simulink library "simeventsrouting1"  (Simulink 7.5)
settings: Solver=ode45  SolverMode=SingleTasking  StartTime=0.0  StopTime=10.0  RelTol=1e-3
undefined symbols (not defined in the file or in its folder): des_support, gcbh
settings Model: Creator=mclune  LastModifiedBy=ywu  ExtModeAutoUpdateStatusClock=off

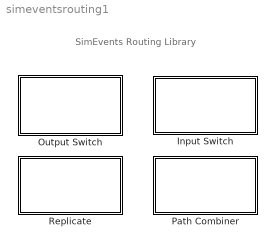
== system simeventsrouting1 ==
  note: SimEvents Routing Library
  Input Switch : Subsystem  Priority=1  LoadFcn=des_support('desLoadFcn',gcbh)  StartFcn=des_support('desStartFcn',gcbh)  StopFcn=des_support('desStopFcn',gcbh)  mask(Input Switch ){NumberInputPorts=3, SwitchingCriterion=Round robin, InitialSeed=23453, SpecifyEventPriority=off, PriorityInputSwitchSelectPort=4000, StatNumberDeparted=Off, StatLastArrivalPort=Off, EvaluatedNumPorts=3}
      mask prompts: NumberInputPorts "Number of entity input ports:"; SwitchingCriterion "Switching criterion:"; InitialSeed "Initial seed:"; SpecifyEventPriority "Resolve simultaneous signal updates according to event priority"; PriorityInputSwitchSelectPort "Event priority:"; StatNumberDeparted "Number of entities departed, #d:"; StatLastArrivalPort "Last entity arrival port, last:"
      mask help:
      | Accept entities from the selected entity input port. The Switching criterion parameter indicates how the block determines which entity input port is selected.
      |
      | The block allows arrivals of entities via exactly one input port. The selected entity input port can change during the simulation. When an entity input port is selected, all others become unavailable.
      mask init:
      | des_inputswitchmask(gcb,'init','apply');
      settings: CopyFcn=des_support('desCopyFcn',gcbh)  DeleteFcn=des_support('desDeleteFcn',gcbh)  UndoDeleteFcn=des_support('desUndoDeleteFcn',gcbh)  ModelCloseFcn=des_support('desModelCloseFcn',gcbh)  PreSaveFcn=des_support('desPreSaveFcn',gcbh)  PostSaveFcn=des_support('desPostSaveFcn',gcbh)  NameChangeFcn=des_support('desNameChangeFcn',gcbh)  CloseFcn=des_support('desCloseFcn',gcbh)  ErrorFcn=des_error_redirect
      mask Help: helpview(simeventsbhelp)
      mask StyleString: edit,popup(Round robin|Equiprobable|From signal port p),edit,checkbox,edit,popup(Off|On|Upon stop or pause),popup(Off|On),edit
      mask CallbackString: des_inputswitchmask(gcb,'cbNumberInputPorts','noapply');|des_inputswitchmask(gcb,'cbSwitchingCriterion','noapply');||des_inputswitchmask(gcb,'cbSpecifyEventPriority','noapply');||des_inputswitchmask(gcb,'cbStatNumberDeparted','noapply');|des_inputswitchmask(gcb,'cbStatLastArrivalPort','noapply');|
      mask TabNameString: Input Switch,Input Switch,Input Switch,Input Switch,Input Switch,Statistics,Statistics,Statistics
      mask Display:
      | image(des_iconLoad('routeSwitchInput.jpg'),'center');
      | port_label('LConn',1,'IN1');
      | port_label('LConn',2,'IN2');
      | port_label('LConn',3,'IN3');
      | port_label('RConn',1,'OUT');
  Output Switch : Subsystem  Priority=1  LoadFcn=des_support('desLoadFcn',gcbh)  StartFcn=des_support('desStartFcn',gcbh)  StopFcn=des_support('desStopFcn',gcbh)  mask(Output Switch){NumberOutputPorts=3, SwitchingCriterion=First port that is not blocked, InitialSeed=34567, AttributeName=Attribute1, InitialConditionsOpt=off, InitialConditions=1, EntityBufferOpt=off, SpecifyEventPriority=off, PriorityOutputSwitchSelectPort=4100, TimeoutPortOpt=off, StatNumberDeparted=Off, StatNumberTimedOut=Off, StatPendingEntity=Off, StatLastDeparturePort=Off, EvaluatedNumPorts=3}
      mask prompts: NumberOutputPorts "Number of entity output ports:"; SwitchingCriterion "Switching criterion:"; InitialSeed "Initial seed:"; AttributeName "Attribute name:"; InitialConditionsOpt "Specify initial port selection"; InitialConditions "Initial port selection:"; EntityBufferOpt "Store entity before switching"; SpecifyEventPriority "Resolve simultaneous signal updates according to event priority"; PriorityOutputSwitchSelectPort "Event priority:"; TimeoutPortOpt "Enable TO port for timed-out entities"; StatNumberDeparted "Number of entities departed, #d:"; StatNumberTimedOut "Number of entities timed out, #to:"; StatPendingEntity "Pending entity present in block, pe:"; StatLastDeparturePort "Last entity departure port, last:"; EvaluatedNumPorts "Evaluated number of ports"
      mask help:
      | Select an entity output port for departure. The Switching criterion parameter indicates how the block determines which entity output port is selected for departure at any given time.
      |
      | The block receives entities and outputs them through one of the entity output ports. The port selected for departures can change during the simulation. When the selected entity output port is not blocked, an arriving entity departs through this port.
      mask init:
      | des_outputswitchmask(gcb,'init','apply')
      settings: CopyFcn=des_support('desCopyFcn',gcbh)  DeleteFcn=des_support('desDeleteFcn',gcbh)  UndoDeleteFcn=des_support('desUndoDeleteFcn',gcbh)  ModelCloseFcn=des_support('desModelCloseFcn',gcbh)  PreSaveFcn=des_support('desPreSaveFcn',gcbh)  PostSaveFcn=des_support('desPostSaveFcn',gcbh)  NameChangeFcn=des_support('desNameChangeFcn',gcbh)  CloseFcn=des_support('desCloseFcn',gcbh)  ErrorFcn=des_error_redirect
      mask Help: helpview(simeventsbhelp)
      mask StyleString: edit,popup(First port that is not blocked|Equiprobable|Round robin|From signal port p|From attribute),edit,edit,checkbox,edit,checkbox,checkbox,edit,checkbox,popup(Off|On|Upon stop or pause),popup(Off|On|Upon stop or pause),popup(Off|On),popup(Off|On),edit
      mask CallbackString: des_outputswitchmask(gcb,'cbNumberOutputPorts','noapply');|des_outputswitchmask(gcb,'cbSwitchingCriterion','noapply');|||des_outputswitchmask(gcb,'cbInitialConditionsOpt','noapply');||des_outputswitchmask(gcb,'cbEntityBufferOpt','noapply');|des_outputswitchmask(gcb,'cbSpecifyEventPriority','noapply');||des_outputswitchmask(gcb,'cbTimeoutPortOpt','noapply');|des_outputswitchmask(gcb,'cbStatNumberDeparted','noapply');|des_outputswitchmask(gcb,'cbStatNumberTimedOut','noapply');|des_outputswitchmask(gcb,'cbStatPendingEntity','noapply');|des_outputswitchmask(gcb,'cbStatLastDeparturePort','noapply');|
      mask TabNameString: Output Switch,Output Switch,Output Switch,Output Switch,Output Switch,Output Switch,Output Switch,Output Switch,Output Switch,Timeout,Statistics,Statistics,Statistics,Statistics,Statistics
      mask Display:
      | image(des_iconLoad('routeSwitchOutput.jpg'),'center');
      | port_label('LConn',1,'IN');
      | port_label('RConn',1,'OUT1');
      | port_label('RConn',2,'OUT2');
      | port_label('RConn',3,'OUT3');
  Path Combiner : Subsystem  Priority=1  LoadFcn=des_support('desLoadFcn',gcbh)  StartFcn=des_support('desStartFcn',gcbh)  StopFcn=des_support('desStopFcn',gcbh)  mask(Path Combiner){NumberInputPorts=3, InputPortPrecedence=IN1 port, InitialSeed=45675, SpecifyEventPriority=off, PriorityPathCombinerPortPrecedenceSelection=4100, StatNumberDeparted=Off, StatLastArrivalPort=Off, EvaluatedNumPorts=3}
      mask prompts: NumberInputPorts "Number of entity input ports:"; InputPortPrecedence "Input port precedence:"; InitialSeed "Initial seed:"; SpecifyEventPriority "Resolve simultaneous signal updates according to event priority"; PriorityPathCombinerPortPrecedenceSelection "Event priority:"; StatNumberDeparted "Number of entities departed, #d:"; StatLastArrivalPort "Last entity arrival port, last:"; EvaluatedNumPorts "Evaluated number of ports"
      mask help:
      | Merge paths, that is, accept entities from any input port and output them through a single entity output port.
      |
      | The Input port precedence parameter indicates how the block determines which entity input port to make available first, whenever the entity output port status changes from blocked to unblocked.
      mask init:
      | des_pathcombinermask(gcb,'init','apply')
      settings: CopyFcn=des_support('desCopyFcn',gcbh)  DeleteFcn=des_support('desDeleteFcn',gcbh)  UndoDeleteFcn=des_support('desUndoDeleteFcn',gcbh)  ModelCloseFcn=des_support('desModelCloseFcn',gcbh)  PreSaveFcn=des_support('desPreSaveFcn',gcbh)  PostSaveFcn=des_support('desPostSaveFcn',gcbh)  NameChangeFcn=des_support('desNameChangeFcn',gcbh)  CloseFcn=des_support('desCloseFcn',gcbh)  ErrorFcn=des_error_redirect
      mask Help: helpview(simeventsbhelp)
      mask StyleString: edit,popup(IN1 port|Equiprobable|Round robin|From signal port p),edit,checkbox,edit,popup(Off|On|Upon stop or pause),popup(Off|On),edit
      mask CallbackString: des_pathcombinermask(gcb,'cbNumberInputPorts','noapply');|des_pathcombinermask(gcb,'cbPortPrecedence','noapply');|des_pathcombinermask(gcb,'cbInitialSeed','noapply');|des_pathcombinermask(gcb,'cbSpecifyEventPriority','noapply');||des_pathcombinermask(gcb,'cbStatNumberDeparted','noapply');|des_pathcombinermask(gcb,'cbStatLastArrivalPort','noapply');|
      mask TabNameString: Path Combiner,Status Notification,Status Notification,Status Notification,Status Notification,Statistics,Statistics,Statistics
      mask Display:
      | image(des_iconLoad('routePathCombine.jpg'),'center');
      | port_label('LConn',1,'IN1');
      | port_label('LConn',2,'IN2');
      | port_label('LConn',3,'IN3');
      | port_label('RConn',1,'OUT');
  Replicate : Subsystem  Priority=1  LoadFcn=des_support('desLoadFcn',gcbh)  StartFcn=des_support('desStartFcn',gcbh)  StopFcn=des_support('desStopFcn',gcbh)  mask(Replicate){NumberOutputPorts=3, ReplicateEntityWhen=All entity output ports are not blocked, OutputPortPrecedence=OUT1 port, InitialSeed=56789, ActionUponBlocking=Discard entity, StatNumberArrived=Off, StatNumberDeparted=Off, EvaluatedNumPorts=3}
      mask prompts: NumberOutputPorts "Number of entity output ports:"; ReplicateEntityWhen "Replicate entity when:"; OutputPortPrecedence "Departure port precedence:"; InitialSeed "Initial seed:"; ActionUponBlocking "If an output port becomes blocked during replication:"; StatNumberArrived "Number of entities arrived, #a:"; StatNumberDeparted "Number of entities departed, #d:"; EvaluatedNumPorts "Evaluated number of ports"
      mask help:
      | Output a copy of the arriving entity through each entity output port that is not blocked.
      |
      | This block accepts an entity to replicate only when the availabilities of subsequent blocks' entity input ports meet the criteria listed in the 'Replicate entity when' parameter.
      mask init:
      | des_replicatemask(gcb,'init','apply')
      settings: CopyFcn=des_support('desCopyFcn',gcbh)  DeleteFcn=des_support('desDeleteFcn',gcbh)  UndoDeleteFcn=des_support('desUndoDeleteFcn',gcbh)  ModelCloseFcn=des_support('desModelCloseFcn',gcbh)  PreSaveFcn=des_support('desPreSaveFcn',gcbh)  PostSaveFcn=des_support('desPostSaveFcn',gcbh)  NameChangeFcn=des_support('desNameChangeFcn',gcbh)  CloseFcn=des_support('desCloseFcn',gcbh)  ErrorFcn=des_error_redirect
      mask Help: helpview(simeventsbhelp)
      mask StyleString: edit,popup(All entity output ports are not blocked|Any entity output port is not blocked),popup(OUT1 port|Round robin|Equiprobable),edit,popup(Discard entity|Warn and discard entity|Error),popup(Off|On|Upon stop or pause),popup(Off|On|Upon stop or pause),edit
      mask CallbackString: des_replicatemask(gcb,'cbNumberOutputPorts','noapply');|des_replicatemask(gcb,'cbReplicateEntityWhen','noapply');|des_replicatemask(gcb,'cbPortPrecedence','noapply');|des_replicatemask(gcb,'cbInitialSeed','noapply');|des_replicatemask(gcb,'cbActionUponBlocking','noapply');|des_replicatemask(gcb,'cbStatNumberArrived','noapply');|des_replicatemask(gcb,'cbStatNumberDeparted','noapply');|
      mask TabNameString: Replicate,Replicate,Replicate,Replicate,Replicate,Statistics,Statistics,Statistics
      mask Display:
      | image(des_iconLoad('routeReplicate.jpg'),'center');
      | port_label('LConn',1,'IN');
      | port_label('RConn',1,'OUT1');
      | port_label('RConn',2,'OUT2');
      | port_label('RConn',3,'OUT3');

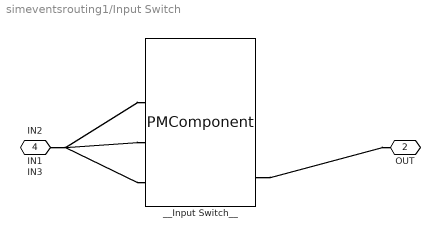
== system simeventsrouting1/Input Switch ==
  __Input Switch__ : PMComponent  PhysicalDomain=simevents  SubClassName=DES_INPUTSWITCH  LeftPortType=desPortIn  RightPortType=desPortOut  LConnTagsString=DI|DI|DI|DI  RConnTagsString=DO|DO|DO
      mask Display:
      | port_label('LConn',1,'p');
      | port_label('LConn',2,'IN1');
      | port_label('LConn',3,'IN2');
      | port_label('LConn',4,'IN3');
      | port_label('RConn',1,'#d');
      | port_label('RConn',2,'last');
      | port_label('RConn',3,'OUT');
  IN1 : PMIOPort  Port=1  Side=Left
  OUT : PMIOPort  Port=2  Side=Right
  IN2 : PMIOPort  Port=3  Side=Left
  IN3 : PMIOPort  Port=4  Side=Left
  connections:
  IN1/RConn1 -- __Input Switch__/LConn2
  __Input Switch__/RConn3 -- OUT/RConn1
  IN2/RConn1 -- __Input Switch__/LConn3
  IN3/RConn1 -- __Input Switch__/LConn4

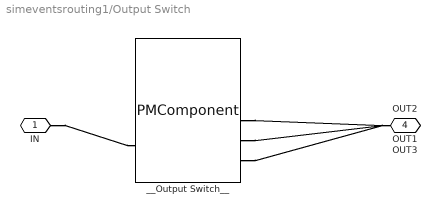
== system simeventsrouting1/Output Switch ==
  __Output Switch__ : PMComponent  PhysicalDomain=simevents  SubClassName=DES_OUTPUTSWITCH  LeftPortType=desPortIn  RightPortType=desPortOut  IconImage=body_sort.jpg  LConnTagsString=DI|DI  RConnTagsString=DO|DO|DO|DO|DO|DO|DO|DO
      mask Display:
      | port_label('LConn',1,'p');
      | port_label('LConn',2,'IN');
      | port_label('RConn',1,'#d');
      | port_label('RConn',2,'#to');
      | port_label('RConn',3,'pe');
      | port_label('RConn',4,'last');
      | port_label('RConn',5,'OUT1');
      | port_label('RConn',6,'OUT2');
      | port_label('RConn',7,'OUT3');
      | port_label('RConn',8,'TO');
  IN : PMIOPort  Port=1  Side=Left
  OUT1 : PMIOPort  Port=2  Side=Right
  OUT2 : PMIOPort  Port=3  Side=Right
  OUT3 : PMIOPort  Port=4  Side=Right
  connections:
  IN/RConn1 -- __Output Switch__/LConn2
  __Output Switch__/RConn5 -- OUT1/RConn1
  __Output Switch__/RConn6 -- OUT2/RConn1
  __Output Switch__/RConn7 -- OUT3/RConn1

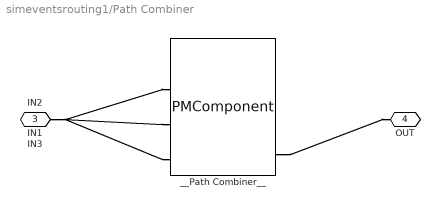
== system simeventsrouting1/Path Combiner ==
  __Path Combiner__ : PMComponent  PhysicalDomain=simevents  SubClassName=DES_PATHCOMBINER  LeftPortType=desPortIn  RightPortType=desPortOut  LConnTagsString=DI|DI|DI|DI  RConnTagsString=DO|DO|DO
      mask Display:
      | port_label('LConn',1,'p');
      | port_label('LConn',2,'IN1');
      | port_label('LConn',3,'IN2');
      | port_label('LConn',4,'IN3');
      | port_label('RConn',1,'#d');
      | port_label('RConn',2,'last');
      | port_label('RConn',3,'OUT');
  IN1 : PMIOPort  Port=1  Side=Left
  IN2 : PMIOPort  Port=2  Side=Left
  IN3 : PMIOPort  Port=3  Side=Left
  OUT : PMIOPort  Port=4  Side=Right
  connections:
  IN1/RConn1 -- __Path Combiner__/LConn2
  IN2/RConn1 -- __Path Combiner__/LConn3
  IN3/RConn1 -- __Path Combiner__/LConn4
  __Path Combiner__/RConn3 -- OUT/RConn1

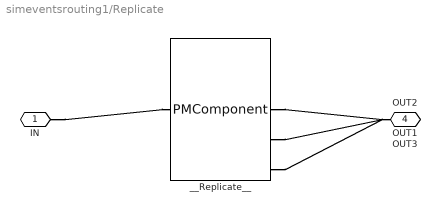
== system simeventsrouting1/Replicate ==
  __Replicate__ : PMComponent  PhysicalDomain=simevents  SubClassName=DES_REPLICATE_ALL  LeftPortType=desPortIn  RightPortType=desPortOut  LConnTagsString=DI  RConnTagsString=DO|DO|DO|DO|DO
      mask Display:
      | port_label('LConn',1,'IN');
      | port_label('RConn',1,'#a');
      | port_label('RConn',2,'#d');
      | port_label('RConn',3,'OUT1');
      | port_label('RConn',4,'OUT2');
      | port_label('RConn',5,'OUT3');
  IN : PMIOPort  Port=1  Side=Left
  OUT1 : PMIOPort  Port=2  Side=Right
  OUT2 : PMIOPort  Port=3  Side=Right
  OUT3 : PMIOPort  Port=4  Side=Right
  connections:
  IN/RConn1 -- __Replicate__/LConn1
  __Replicate__/RConn3 -- OUT1/RConn1
  __Replicate__/RConn4 -- OUT2/RConn1
  __Replicate__/RConn5 -- OUT3/RConn1
